simulink model "Bioreactor2_arduino_Conexion"  (R2016a)
settings: Solver=VariableStepAuto  StartTime=0.0  StopTime=3000  RelTol=1e-3
libraries: instrumentlib x2
settings Model: Creator=Daniel  LastModifiedBy=Daniel

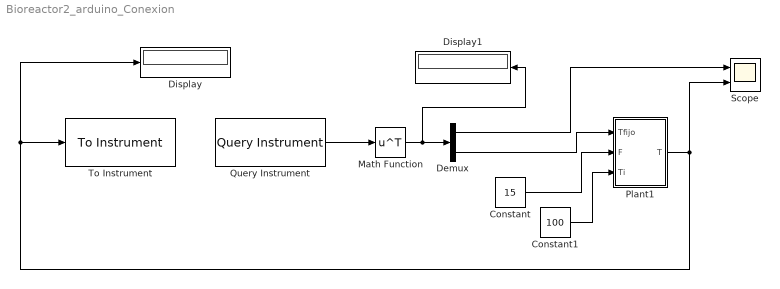
== system Bioreactor2_arduino_Conexion ==
  Constant : Constant  Value=15
  Constant1 : Constant  Value=100
  Demux : Demux  Outputs=2
  Display : Display
  Display1 : Display
  Math Function : Math  Operator=transpose  SaturateOnIntegerOverflow=on
  Plant1 : Subsystem
  Query Instrument : instrumentlib/Query Instrument  sampleTime=4  isWorkspaceObject=off  timeout=10  inputBufferSize=512  protocol=Serial  serialPort=COM3  baudRate=9600  gpibVendor=Agilent Technologies  boardIndex=0  primaryAddress=1  secondaryAddress=0  visaVendor=Agilent  visaSerialPort=0  chassisIndex=0  logicalAddress=0  tcpRemoteHost='127.0.0.1'  tcpRemotePort=4500  udpRemoteHost='127.0.0.1'  udpRemotePort=9090  visaTCPBoardIndex=0  visaTCPRemoteHost='127.0.0.1'  usbBoardIndex=0  usbManufID=0  usbModelCode=0  usbSerialNumber=0  initAction=None  initCommand='DATA:SOURCE CH1'  initFunction=get  queryCommand='curve?'  responseFormat=ASCII  asciiFormatting='%f,%f'  precision=8-bit integer  byteOrder=Little Endian  valuesToRead=1  removeBytes=off  afterOutputAction=Repeat query for new data  enableFrames=on  frameSize=2
  Scope : Scope  NumInputPorts=2
  To Instrument : instrumentlib/To Instrument  sampleTime=4  isWorkspaceObject=off  timeout=10  inputBufferSize=8192  protocol=Serial  serialPort=COM3  baudRate=9600  gpibVendor=Agilent Technologies  boardIndex=0  primaryAddress=1  secondaryAddress=0  visaVendor=Agilent  visaSerialPort=0  chassisIndex=0  logicalAddress=0  tcpRemoteHost='127.0.0.1'  tcpRemotePort=4500  udpRemoteHost='127.0.0.1'  udpRemotePort=9090  visaTCPBoardIndex=0  visaTCPRemoteHost='127.0.0.1'  usbBoardIndex=0  usbManufID=0  usbModelCode=0  usbSerialNumber=0  initAction=None  initCommand='DATA:SOURCE CH1'  initFunction=get  command=''  sendFormat=ASCII  asciiFormatting='%f'  precision=8-bit integer  byteOrder=Little Endian
  wires:
  Plant1/1(T) -> To Instrument/1, Display/1, Scope/2
  Demux/1 -> Scope/1
  Query Instrument/1 -> Math Function/1
  Math Function/1 -> Demux/1, Display1/1
  Constant1/1 -> Plant1/3(Ti)
  Constant/1 -> Plant1/2(F)
  Demux/2 -> Plant1/1(Tfijo)

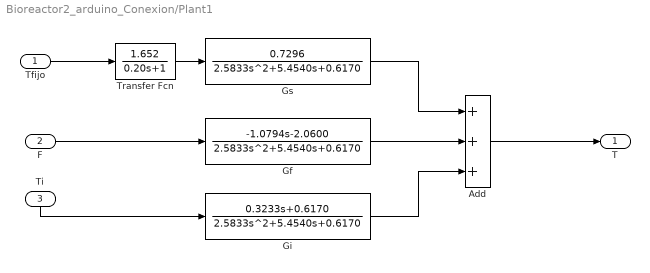
== system Bioreactor2_arduino_Conexion/Plant1 ==
  Tfijo : Inport
  F : Inport  Port=2
  Ti : Inport  Port=3
  Add : Sum  Inputs=+++
  Gf : TransferFcn  Numerator=[-1.0794 -2.0600]  Denominator=[2.5833 5.4540 0.6170]
  Gi : TransferFcn  Numerator=[0.3233 0.6170]  Denominator="[2.5833 5.4540  0.6170]"
  Gs : TransferFcn  Numerator=[0.7296]  Denominator="[2.5833 5.4540  0.6170]"
  Transfer Fcn : TransferFcn  Numerator=[1.652]  Denominator=[0.20 1]
  T : Outport
  wires:
  Add/1 -> T/1
  Gi/1 -> Add/3
  Gf/1 -> Add/2
  Transfer Fcn/1 -> Gs/1
  Gs/1 -> Add/1
  Ti/1 -> Gi/1
  Tfijo/1 -> Transfer Fcn/1
  F/1 -> Gf/1
